simulink library "ESTS_FRIC_HILO_CONDLOG"  (R2024b)
settings: Solver=VariableStepAuto  StartTime=0.0  StopTime=10.0  RelTol=1e-3
settings Model: Creator=blatak  LastModifiedBy=blatak

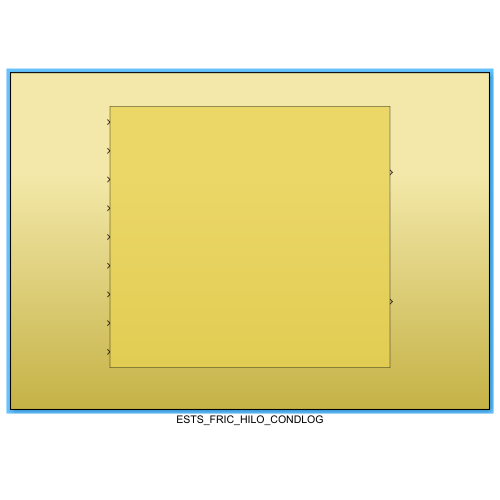
[thumbnail: Simulink's stored preview of the top-level diagram]
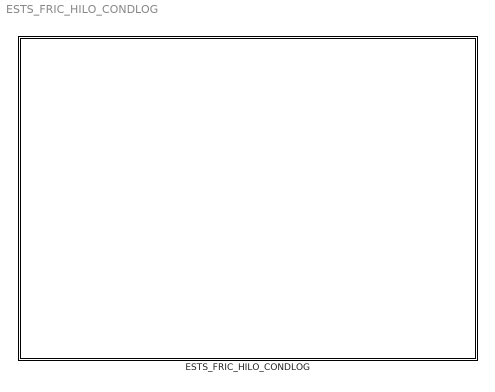
== system ESTS_FRIC_HILO_CONDLOG ==
  ESTS_FRIC_HILO_CONDLOG : Subsystem

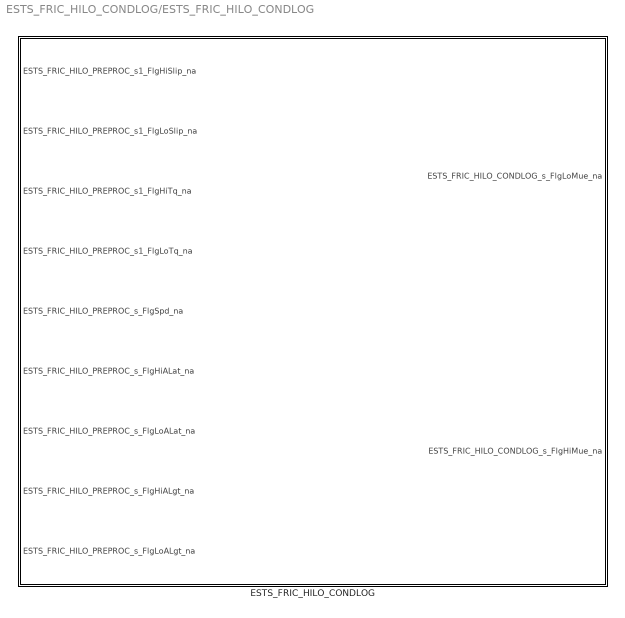
== system ESTS_FRIC_HILO_CONDLOG/ESTS_FRIC_HILO_CONDLOG ==
  ESTS_FRIC_HILO_CONDLOG : Subsystem

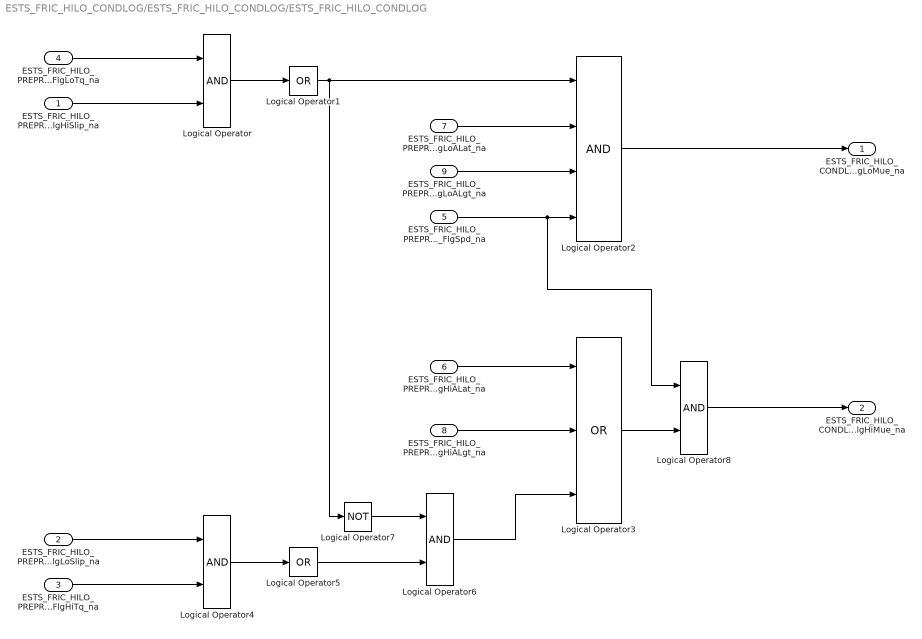
== system ESTS_FRIC_HILO_CONDLOG/ESTS_FRIC_HILO_CONDLOG/ESTS_FRIC_HILO_CONDLOG ==
  ESTS_FRIC_HILO_PREPROC_s1_FlgHiSlip_na : Inport
  ESTS_FRIC_HILO_PREPROC_s1_FlgLoSlip_na : Inport  Port=2
  ESTS_FRIC_HILO_PREPROC_s1_FlgHiTq_na : Inport  Port=3
  ESTS_FRIC_HILO_PREPROC_s1_FlgLoTq_na : Inport  Port=4
  ESTS_FRIC_HILO_PREPROC_s_FlgSpd_na : Inport  Port=5
  ESTS_FRIC_HILO_PREPROC_s_FlgHiALat_na : Inport  Port=6
  ESTS_FRIC_HILO_PREPROC_s_FlgLoALat_na : Inport  Port=7
  ESTS_FRIC_HILO_PREPROC_s_FlgHiALgt_na : Inport  Port=8
  ESTS_FRIC_HILO_PREPROC_s_FlgLoALgt_na : Inport  Port=9
  Logical Operator{,4,6,8} (4 alike) : Logic  AllPortsSameDT=off  OutDataTypeStr=boolean
  Logical Operator1 : Logic  Operator=OR  Inputs=1  AllPortsSameDT=off  OutDataTypeStr=boolean
  Logical Operator2 : Logic  Inputs=4  AllPortsSameDT=off  OutDataTypeStr=boolean
  Logical Operator3 : Logic  Operator=OR  Inputs=3  AllPortsSameDT=off  OutDataTypeStr=boolean
  Logical Operator5 : Logic  Operator=OR  Inputs=1  AllPortsSameDT=off  OutDataTypeStr=boolean
  Logical Operator7 : Logic  Operator=NOT  AllPortsSameDT=off  OutDataTypeStr=boolean
  ESTS_FRIC_HILO_CONDLOG_s_FlgLoMue_na : Outport
  ESTS_FRIC_HILO_CONDLOG_s_FlgHiMue_na : Outport  Port=2
  wires:
  Logical Operator4/1 -> Logical Operator5/1
  ESTS_FRIC_HILO_PREPROC_s1_FlgLoSlip_na/1 -> Logical Operator4/1
  ESTS_FRIC_HILO_PREPROC_s_FlgSpd_na/1 -> Logical Operator8/1, Logical Operator2/4
  ESTS_FRIC_HILO_PREPROC_s1_FlgHiSlip_na/1 -> Logical Operator/2
  ESTS_FRIC_HILO_PREPROC_s1_FlgLoTq_na/1 -> Logical Operator/1
  Logical Operator1/1 -> Logical Operator7/1, Logical Operator2/1
  ESTS_FRIC_HILO_PREPROC_s_FlgLoALgt_na/1 -> Logical Operator2/3
  Logical Operator3/1 -> Logical Operator8/2
  Logical Operator8/1 -> ESTS_FRIC_HILO_CONDLOG_s_FlgHiMue_na/1
  ESTS_FRIC_HILO_PREPROC_s_FlgLoALat_na/1 -> Logical Operator2/2
  ESTS_FRIC_HILO_PREPROC_s_FlgHiALgt_na/1 -> Logical Operator3/2
  ESTS_FRIC_HILO_PREPROC_s_FlgHiALat_na/1 -> Logical Operator3/1
  Logical Operator7/1 -> Logical Operator6/1
  Logical Operator2/1 -> ESTS_FRIC_HILO_CONDLOG_s_FlgLoMue_na/1
  Logical Operator/1 -> Logical Operator1/1
  Logical Operator6/1 -> Logical Operator3/3
  Logical Operator5/1 -> Logical Operator6/2
  ESTS_FRIC_HILO_PREPROC_s1_FlgHiTq_na/1 -> Logical Operator4/2
